simulink model "sldemo_variant_subsystems"  (Simulink 10.0)
settings: Solver=FixedStepDiscrete  StartTime=0.0  StopTime=10.0  RelTol=1e-3  EnableMultiTasking=on
PreLoadFcn:
  | VSS_LINEAR_CONTROLLER=Simulink.Variant('VSS_MODE==1')
  | VSS_NONLINEAR_CONTROLLER=Simulink.Variant('VSS_MODE==2')
  | 
  | VSS_MODE=2
Description:
  | Variant Subsystems
  | 
  | This model illustrates Simulink(R) variant subsystems. Variant subsystems let
  | you provide multiple implementations to a subsystem where only one
  | implementation is active during simulation. You can programmatically swap out
  | the active implementation and replace it with one of the other implementations
  | without modifying the model.
settings Model: FPTRunName=Active  Creator=The MathWorks, Inc.  LastModifiedBy=bhisma
settings DataIOCC: LimitDataPoints=on  ReturnWorkspaceOutputs=on
settings OptimizationCC: DefaultParameterBehavior=Inlined  ExpressionDepthLimit=2147483647
settings DebuggingCC: UnderspecifiedInitializationDetection=Simplified  MergeDetectMultiDrivingBlocksExec=error  SolverPrmCheckMsg=warning  FcnCallInpInsideContextMsg=warning  StateNameClashWarn=warning
settings GRTTargetCC: GeneratePreprocessorConditionals=Disable all
settings ConfigComp: CovExternalEMLEnable=off  CovSFcnEnable=off

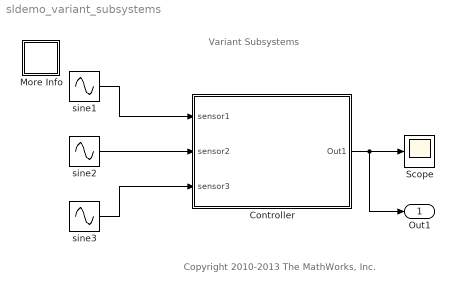
== system sldemo_variant_subsystems ==
  note: Copyright 2010-2013 The MathWorks, Inc.
  note: Variant Subsystems
  Controller : Subsystem  Variant=on
  More Info : Subsystem
      settings: OpenFcn=showdemo(bdroot(gcb))
      mask Display: disp('?')
  Scope : Scope
  sine1 : Sin  Amplitude=.1  Frequency=pi/3  SampleTime=.01
  sine2 : Sin  Amplitude=2  SampleTime=.01
  sine3 : Sin  Amplitude=.3  Frequency=pi/6  SampleTime=.01
  Out1 : Outport  VectorParamsAs1DForOutWhenUnconnected=off
  wires:
  sine2/1 -> Controller/2(sensor2)
  sine1/1 -> Controller/1(sensor1)
  sine3/1 -> Controller/3(sensor3)
  Controller/1(Out1) -> Scope/1, Out1/1

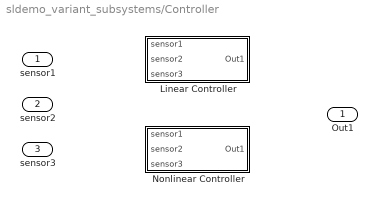
== system sldemo_variant_subsystems/Controller ==
  sensor1 : Inport
  sensor2 : Inport  Port=2
  sensor3 : Inport  Port=3
  Linear Controller : Subsystem  VariantControl=VSS_LINEAR_CONTROLLER
  Nonlinear Controller : Subsystem  VariantControl=VSS_NONLINEAR_CONTROLLER
  Out1 : Outport  VectorParamsAs1DForOutWhenUnconnected=off

== system sldemo_variant_subsystems/More Info ==
  note: This model illustrates Simulink variant subsystems. Variant subsystems let you
      | provide multiple implementations for a subsystem where only one
      | implementation is active during simulation. You can programmatically swap out
      | the active implementation and replace it with one of the other implementations
      | without modifying the model.
  note: Variant Subsystems

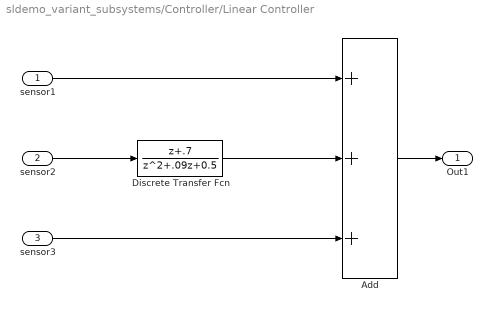
== system sldemo_variant_subsystems/Controller/Linear Controller ==
  sensor1 : Inport
  sensor2 : Inport  Port=2
  sensor3 : Inport  Port=3
  Add : Sum  Inputs=+++
  Discrete Transfer Fcn : DiscreteTransferFcn  Numerator=[1 .7]  Denominator=[1 .09 0.5]  SampleTime=.01
  Out1 : Outport  VectorParamsAs1DForOutWhenUnconnected=off
  wires:
  sensor2/1 -> Discrete Transfer Fcn/1
  Discrete Transfer Fcn/1 -> Add/2
  sensor3/1 -> Add/3
  sensor1/1 -> Add/1
  Add/1 -> Out1/1

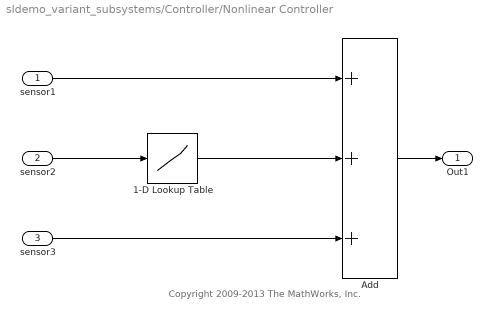
== system sldemo_variant_subsystems/Controller/Nonlinear Controller ==
  note: Copyright 2009-2013 The MathWorks, Inc.
  sensor1 : Inport
  sensor2 : Inport  Port=2
  sensor3 : Inport  Port=3
  1-D Lookup Table : Lookup_n-D  NumberOfTableDimensions=1  BreakpointsForDimension1=[-5:5]  Table=tanh([-5:5])  InputSameDT=on
  Add : Sum  Inputs=+++  SampleTime=.01
  Out1 : Outport  VectorParamsAs1DForOutWhenUnconnected=off
  wires:
  sensor2/1 -> 1-D Lookup Table/1
  1-D Lookup Table/1 -> Add/2
  sensor3/1 -> Add/3
  sensor1/1 -> Add/1
  Add/1 -> Out1/1
